simulink model "c1_f"  (R2021b)
settings: Solver=VariableStepAuto  StartTime=0.0  StopTime=10  RelTol=1e-3
settings Model: Creator=Studenci  LastModifiedBy=Studenci

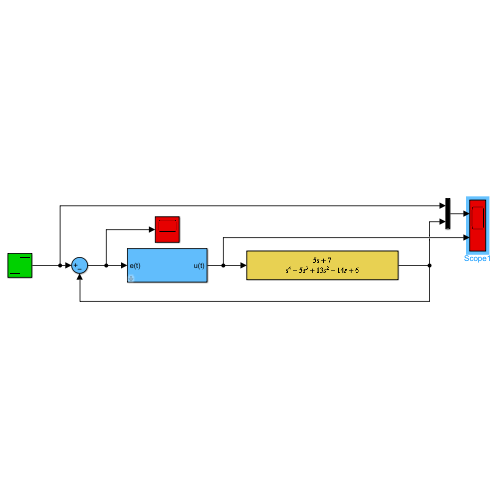
[thumbnail: Simulink's stored preview of the top-level diagram]
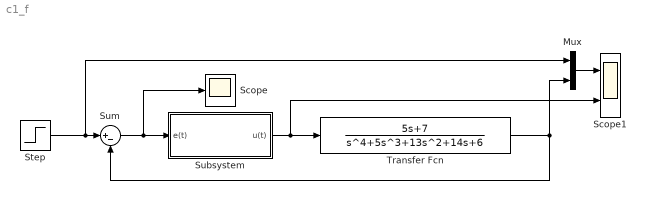
== system c1_f ==
  Mux : Mux  Inputs=2
  Scope : Scope
  Scope1 : Scope  NumInputPorts=2
  Step : Step  Time=0  SampleTime=0
  Subsystem : Subsystem  mask{Kp=2.972367437761131, Ki=2.634595834216244, Kd=0.838360866429722}
      mask prompts: Kp "Kp ="; Ki "Ki ="; Kd "Kd ="
  Sum : Sum  Inputs=|+-
  Transfer Fcn : TransferFcn  Numerator=[5 7]  Denominator=[1 5 13 14 6]
  wires:
  Step/1 -> Mux/1, Sum/1
  Sum/1 -> Subsystem/1(e(t)), Scope/1
  Subsystem/1(u(t)) -> Scope1/2, Transfer Fcn/1
  Mux/1 -> Scope1/1
  Transfer Fcn/1 -> Sum/2, Mux/2

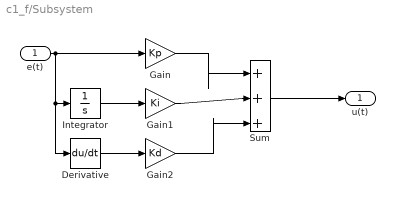
== system c1_f/Subsystem ==
  e(t) : Inport
  Derivative : Derivative
  Gain : Gain  Gain=Kp
  Gain1 : Gain  Gain=Ki
  Gain2 : Gain  Gain=Kd
  Integrator : Integrator
  Sum : Sum  Inputs=|+++
  u(t) : Outport
  wires:
  Integrator/1 -> Gain1/1
  e(t)/1 -> Derivative/1, Integrator/1, Gain/1
  Gain/1 -> Sum/1
  Gain1/1 -> Sum/2
  Gain2/1 -> Sum/3
  Sum/1 -> u(t)/1
  Derivative/1 -> Gain2/1
